simulink model "VRSimulationModel"  (R2020b)
settings: Solver=VariableStepAuto  StartTime=0.0  StopTime=30  RelTol=1e-3
undefined symbols (not defined in the file): cz_length, lane_width
libraries: drivingvehiclecontroller x4, etargetslib x2, rllib x2, dspnetwork x2
settings Model: EnablePacing=on  Creator=ZHANG Meng  LastModifiedBy=ZHANG Meng

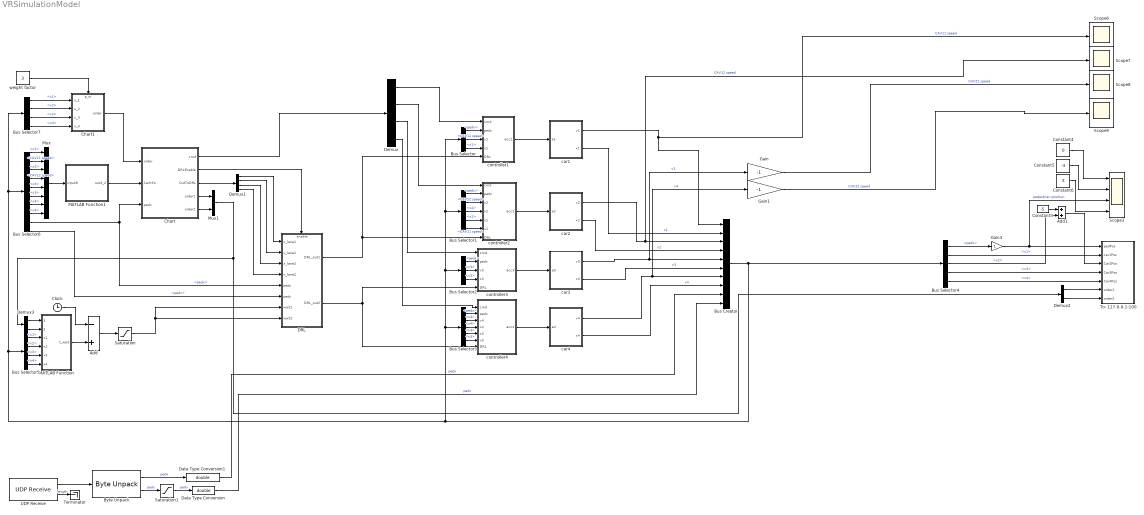
== system VRSimulationModel ==
  Add : Sum  Inputs=-+
  Add1 : Sum
  Bus Creator : BusCreator  Inputs=10
  Bus Selector : BusSelector  OutputSignals=pedx,CAV11 speed,x1
  Bus Selector1 : BusSelector  OutputSignals=pedx,CAV12 speed,x2,x1,CAV11 speed
  Bus Selector2 : BusSelector  OutputSignals=pedx,v3,x3
  Bus Selector3 : BusSelector  OutputSignals=pedx,v4,x4,x3,v3
  Bus Selector4 : BusSelector  OutputSignals=pedx,x1,x2,x3,x4
  Bus Selector5 : BusSelector  OutputSignals=x1,x2,x3,x4
  Bus Selector6 : BusSelector  OutputSignals=x1,CAV11 speed,x2,CAV12 speed,x3,v3,x4,v4,pedx,pedv
  Bus Selector7 : BusSelector  OutputSignals=x1,x2,x3,x4
  Byte Unpack : etargetslib/Byte Unpack  dimensions={1,1}  datatypes={'single','single'}  byteAlign=1
  Chart : Stateflow chart  TreatAsAtomicUnit=on
  Chart1 : Stateflow chart  TreatAsAtomicUnit=on
      settings: PortSchema="{\"entries\":[{\"content\":{\"sides\":[{\"content\":{\"connectorIds\":[\"In1\",\"In2\",\"In3\",\"In4\"]},\"type\":\"ConnectorPlacement.EquallySpacedRectSide\",\"uuid\":\"8a846dc3-1f93-46d5-8c0a-752417c681d9\"},{\"content\":{\"connectorIds\":[\"Out1\"],\"side\":\"RIGHT\"},\"type\":\"ConnectorPlacement.EquallySpacedRectSide\",\"uuid\":\"76ec7057-478a-4564-adde-c35c4c2d4bf9\"},{\"content\":{\"connectorIds\":[\"In5\"],\"side\":\"TOP\"},\"type\":\"ConnectorPlacement.EquallySpacedRectSide\",\"uuid\":\"bd3b034c-69d7-410c-9bea-d641b8557378\"}]},\"type\":\"ConnectorPlacement.EquallySpacedConnector\",\"uuid\":\"e6d2d864-1dd5-4aa2-85d9-3c27811e9247\"}],\"packageUris\":[\"http://schema.mathworks.com/mf0/Connector/R2020b\"],\"version\":\"1.0\"}"
  Clock : Clock
  Constant3 : Constant  Value=-5
  Constant4 : Constant  Value=0
  Constant5 : Constant  Value=-3
  Constant6 : Constant  Value=3
  DRL : Subsystem  TreatAsAtomicUnit=on
  Data Type Conversion : DataTypeConversion  OutDataTypeStr=double
  Data Type Conversion1 : DataTypeConversion  OutDataTypeStr=double
  Demux : Demux
  Demux1 : Demux
  Demux2 : Demux  Outputs=2
  Demux3 : Demux  Outputs=2
  Gain : Gain  Gain=-1
  Gain1 : Gain  Gain=-1
  Gain3 : Gain
  MATLAB Function : MATLAB Function  TreatAsAtomicUnit=on
  MATLAB Function1 : MATLAB Function  TreatAsAtomicUnit=on
  Mux : Mux  Inputs=8
  Mux1 : Mux  Inputs=2
  Saturation : Saturate  UpperLimit=20  LowerLimit=0
  Saturation1 : Saturate  UpperLimit=2  LowerLimit=0
  Scope3 : Scope  NumInputPorts=4
  Scope{6..9} (4 alike) : Scope
  Terminator : Terminator
  To: 127.0.0.1:100 : Subsystem
  UDP Receive : dspnetwork/UDP Receive  localURL='0.0.0.0'  localPort=200  remoteURL='127.0.0.1'  remotePort=-1  recvBufferSize=100  dims=8  signalDatatype=uint8  isComplex=off  isVarSize=off  showBlockingTime=off  blockingTime=0  sampletime=0.1  blockPlatform=[]
  car1 : Subsystem
  car2 : Subsystem
  car3 : Subsystem
  car4 : Subsystem
  controller1 : Subsystem
  controller2 : Subsystem
  controller3 : Subsystem
  controller4 : Subsystem
  weight factor : Constant  Value=3
  wires:
  controller4/1(acc4) -> car4/1(a4)
  controller2/1(acc2) -> car2/1(a2)
  controller3/1(acc3) -> car3/1(a3)
  car1/1(v1) -> Scope6/1, Bus Creator/1  "CAV11 speed"
  car1/2(x1) -> Bus Creator/2  "x1"
  car2/1(v2) -> Scope7/1, Bus Creator/3  "CAV12 speed"
  car2/2(x2) -> Bus Creator/4  "x2"
  car3/1(v3) -> Gain/1, Bus Creator/5  "v3"
  car3/2(x3) -> Bus Creator/6  "x3"
  car4/1(v4) -> Gain1/1, Bus Creator/7  "v4"
  car4/2(x4) -> Bus Creator/8  "x4"
  Bus Creator/1 -> Bus Selector4/1, Bus Selector1/1, Bus Selector/1, Bus Selector2/1, Bus Selector3/1, Bus Selector7/1, Bus Selector6/1, Bus Selector5/1
  Bus Selector/2 -> controller1/3(v1)  "<CAV11 speed>"
  Bus Selector/1 -> controller1/2(pedx)  "<pedx>"
  Bus Selector/3 -> controller1/4(x1)  "<x1>"
  Bus Selector1/5 -> controller2/6(v1)  "<CAV11 speed>"
  Bus Selector1/4 -> controller2/5(x1)  "<x1>"
  Bus Selector1/3 -> controller2/4(x2)  "<x2>"
  Bus Selector1/2 -> controller2/3(v2)  "<CAV12 speed>"
  Bus Selector1/1 -> controller2/2(pedx)  "<pedx>"
  Bus Selector2/1 -> controller3/2(pedx)  "<pedx>"
  Bus Selector2/2 -> controller3/3(v3)  "<v3>"
  Bus Selector2/3 -> controller3/4(x3)  "<x3>"
  Bus Selector3/1 -> controller4/2(pedx)  "<pedx>"
  Bus Selector3/2 -> controller4/3(v4)  "<v4>"
  Bus Selector3/3 -> controller4/4(x4)  "<x4>"
  Bus Selector3/4 -> controller4/5(x3)  "<x3>"
  Bus Selector3/5 -> controller4/6(v3)  "<v3>"
  Demux/4 -> controller4/1(cmd)
  Gain/1 -> Scope8/1  "CAV21 speed"
  Demux/2 -> controller2/1(cmd)
  Gain1/1 -> Scope9/1  "CAV22 speed"
  Demux/3 -> controller3/1(cmd)
  Demux/1 -> controller1/1(cmd)
  Chart/1(cmd) -> Demux/1
  Bus Selector6/8 -> Mux/8  "<v4>"
  Bus Selector6/7 -> Mux/7  "<x4>"
  Bus Selector6/5 -> Mux/5  "<x3>"
  Bus Selector6/6 -> Mux/6  "<v3>"
  Bus Selector6/4 -> Mux/4  "<CAV12 speed>"
  Bus Selector6/3 -> Mux/3  "<x2>"
  Bus Selector6/2 -> Mux/2  "<CAV11 speed>"
  Bus Selector6/1 -> Mux/1  "<x1>"
  Mux/1 -> MATLAB Function1/1(input8)
  MATLAB Function1/1(out4_2) -> Chart/2(CarInfo)
  Bus Selector6/9 -> DRL/5(pedx), Chart/3(pedx)  "<pedx>"
  Chart/3(OutToDRL) -> Demux1/1
  Chart/2(DRLEnable) -> DRL/Enable
  Demux1/1 -> DRL/1(x_lane1)
  Demux1/2 -> DRL/2(v_lane1)
  Demux1/3 -> DRL/3(x_lane2)
  Demux1/4 -> DRL/4(v_lane2)
  Bus Selector6/10 -> DRL/6(pedv)  "<pedv>"
  Bus Selector7/1 -> Chart1/1(x_1)  "<x1>"
  Bus Selector7/2 -> Chart1/2(x_2)  "<x2>"
  Bus Selector7/3 -> Chart1/3(x_3)  "<x3>"
  Bus Selector7/4 -> Chart1/4(x_4)  "<x4>"
  Chart1/1(order) -> Chart/1(order)
  weight factor/1 -> Chart1/5(p_w)
  controller1/1(acc1) -> car1/1(a1)
  DRL/1(DRL_out1) -> controller2/7(DRL), controller1/5(DRL)
  DRL/2(DRL_out2) -> controller4/7(DRL), controller3/5(DRL)
  Saturation/1 -> DRL/7(wait1), DRL/8(wait2)
  Add/1 -> Saturation/1
  MATLAB Function/1(t_wait) -> Add/2
  Clock/1 -> Add/1
  Gain3/1 -> Scope3/3, To: 127.0.0.1:100/1(pedPos)  "pedestrian position"
  Bus Selector4/1 -> Gain3/1  "<pedx>"
  Bus Selector4/5 -> To: 127.0.0.1:100/5(Car4Pos)  "<x4>"
  Constant4/1 -> Scope3/1
  Constant5/1 -> Scope3/2
  Constant6/1 -> Scope3/4
  Chart/4(order1) -> Mux1/1
  Chart/5(order2) -> Mux1/2
  Demux2/1 -> To: 127.0.0.1:100/6(order1)
  Demux2/2 -> To: 127.0.0.1:100/7(order2)
  Mux1/1 -> Demux3/1, Demux2/1
  UDP Receive/1 -> Byte Unpack/1
  Saturation1/1 -> Data Type Conversion/1  "pedv"
  Data Type Conversion1/1 -> Bus Creator/9  "pedx"
  Data Type Conversion/1 -> Bus Creator/10  "pedv"
  Bus Selector5/1 -> MATLAB Function/3(x1)  "<x1>"
  Bus Selector5/2 -> MATLAB Function/4(x2)  "<x2>"
  Bus Selector5/3 -> MATLAB Function/5(x3)  "<x3>"
  Bus Selector5/4 -> MATLAB Function/6(x4)  "<x4>"
  Demux3/1 -> MATLAB Function/1(order1)
  Demux3/2 -> MATLAB Function/2(order2)
  Constant3/1 -> Add1/1
  Bus Selector4/2 -> To: 127.0.0.1:100/2(car1Pos)  "<x1>"
  Bus Selector4/4 -> To: 127.0.0.1:100/4(Car3Pos)  "<x3>"
  Bus Selector4/3 -> Add1/2  "<x2>"
  Add1/1 -> To: 127.0.0.1:100/3(Car2Pos)
  UDP Receive/2 -> Terminator/1  "length"
  Byte Unpack/1 -> Data Type Conversion1/1  "pedx"
  Byte Unpack/2 -> Saturation1/1  "pedv"

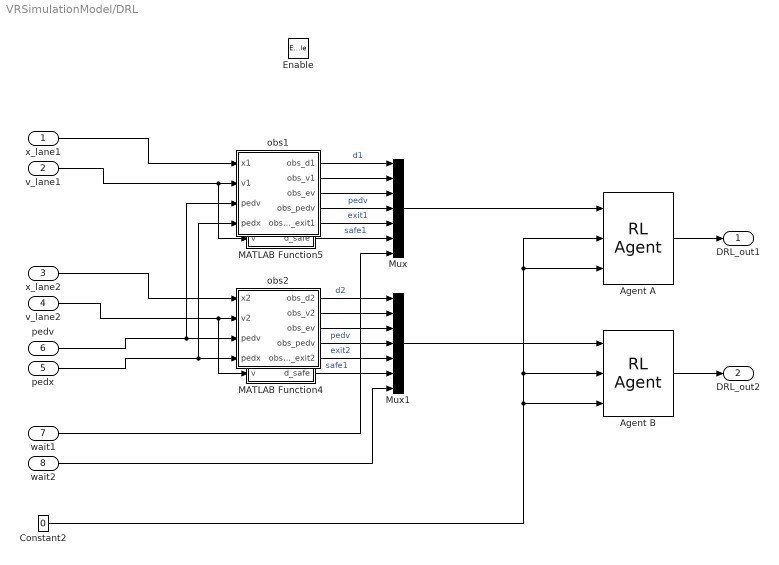
== system VRSimulationModel/DRL ==
  x_lane1 : Inport
  v_lane1 : Inport  Port=2
  x_lane2 : Inport  Port=3
  v_lane2 : Inport  Port=4
  pedx : Inport  Port=5
  pedv : Inport  Port=6
  wait1 : Inport  Port=7
  wait2 : Inport  Port=8
  Enable : EnablePort
  Agent A : rllib/RL Agent  Agent=agentA  ProvideReward=on  ProvideIsDone=on  ProvideCumRwd=off  TreatAsDirectFeedthrough=on  CollectLoggedSignals=on  CollectModelStates=on
  Agent B : rllib/RL Agent  Agent=agentB  ProvideReward=on  ProvideIsDone=on  ProvideCumRwd=off  TreatAsDirectFeedthrough=on  CollectLoggedSignals=on  CollectModelStates=on
  Constant2 : Constant  Value=0
  MATLAB Function4 : MATLAB Function  TreatAsAtomicUnit=on
  MATLAB Function5 : MATLAB Function  TreatAsAtomicUnit=on
  Mux : Mux  Inputs=7
  Mux1 : Mux  Inputs=7
  obs1 : Subsystem
  obs2 : Subsystem
  DRL_out1 : Outport
  DRL_out2 : Outport  Port=2
  wires:
  Constant2/1 -> Agent A/2, Agent A/3, Agent B/2, Agent B/3
  x_lane1/1 -> obs1/1(x1)
  x_lane2/1 -> obs2/1(x2)
  v_lane1/1 -> MATLAB Function5/1(v), obs1/2(v1)
  pedx/1 -> obs1/4(pedx), obs2/4(pedx)
  pedv/1 -> obs1/3(pedv), obs2/3(pedv)
  Agent B/1 -> DRL_out2/1
  Agent A/1 -> DRL_out1/1
  v_lane2/1 -> MATLAB Function4/1(v), obs2/2(v2)
  obs1/1(obs_d1) -> Mux/1  "d1"
  obs1/2(obs_v1) -> Mux/2
  obs1/3(obs_ev) -> Mux/3
  obs1/4(obs_pedv) -> Mux/4  "pedv"
  obs1/5(obs_d_exit1) -> Mux/5  "exit1"
  MATLAB Function5/1(d_safe) -> Mux/6  "safe1"
  obs2/2(obs_v2) -> Mux1/2
  obs2/4(obs_pedv) -> Mux1/4  "pedv"
  obs2/3(obs_ev) -> Mux1/3
  obs2/1(obs_d2) -> Mux1/1  "d2"
  obs2/5(obs_d_exit2) -> Mux1/5  "exit2"
  MATLAB Function4/1(d_safe) -> Mux1/6  "safe1"
  Mux/1 -> Agent A/1
  Mux1/1 -> Agent B/1
  wait1/1 -> Mux/7
  wait2/1 -> Mux1/7

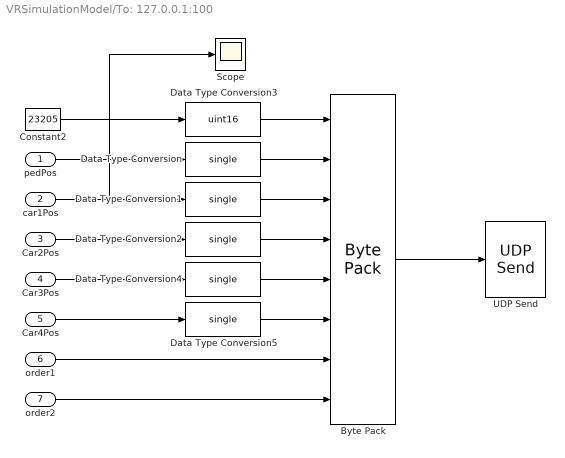
== system VRSimulationModel/To: 127.0.0.1:100 ==
  pedPos : Inport
  car1Pos : Inport  Port=2
  Car2Pos : Inport  Port=3
  Car3Pos : Inport  Port=4
  Car4Pos : Inport  Port=5
  order1 : Inport  Port=6
  order2 : Inport  Port=7
  Byte Pack : etargetslib/Byte Pack  datatypes={'uint16','single','single','single','single','single','uint8','uint8'}  byteAlign=1
  Constant2 : Constant  Value=23205  SampleTime=0.02
  Data Type Conversion{,1..2,4..5} (5 alike) : DataTypeConversion  OutDataTypeStr=single
  Data Type Conversion3 : DataTypeConversion  OutDataTypeStr=uint16
  Scope : Scope
  UDP Send : dspnetwork/UDP Send  remoteURL='127.0.0.1'  remotePort=100  localURL='0.0.0.0'  localPortSource=Specify via dialog  localPort=300  sendBufferSize=200  sampletime=-1  blockPlatform=[]  separateLengthPort=0
  wires:
  Data Type Conversion3/1 -> Byte Pack/1
  Byte Pack/1 -> UDP Send/1
  Constant2/1 -> Data Type Conversion3/1
  car1Pos/1 -> Scope/1, Data Type Conversion1/1
  Data Type Conversion1/1 -> Byte Pack/3
  Data Type Conversion/1 -> Byte Pack/2
  Data Type Conversion2/1 -> Byte Pack/4
  pedPos/1 -> Data Type Conversion/1
  Car2Pos/1 -> Data Type Conversion2/1
  Car4Pos/1 -> Data Type Conversion5/1
  Car3Pos/1 -> Data Type Conversion4/1
  Data Type Conversion4/1 -> Byte Pack/5
  Data Type Conversion5/1 -> Byte Pack/6
  order1/1 -> Byte Pack/7
  order2/1 -> Byte Pack/8

== system VRSimulationModel/car1 ==
  a1 : Inport
  Integrator : Integrator  InitialCondition=10  LimitOutput=on  LowerSaturationLimit=0
  Integrator1 : Integrator  InitialCondition=-30
  Transfer Fcn : TransferFcn  Denominator=[0.2 1]
  v1 : Outport
  x1 : Outport  Port=2
  wires:
  a1/1 -> Transfer Fcn/1
  Integrator/1 -> v1/1, Integrator1/1
  Transfer Fcn/1 -> Integrator/1
  Integrator1/1 -> x1/1

== system VRSimulationModel/car2 ==
  a2 : Inport
  Integrator : Integrator  InitialCondition=10  LimitOutput=on  LowerSaturationLimit=0
  Integrator1 : Integrator  InitialCondition=-75
  Transfer Fcn : TransferFcn  Denominator=[0.2 1]
  v2 : Outport
  x2 : Outport  Port=2
  wires:
  a2/1 -> Transfer Fcn/1
  Integrator/1 -> v2/1, Integrator1/1
  Transfer Fcn/1 -> Integrator/1
  Integrator1/1 -> x2/1

== system VRSimulationModel/car3 ==
  a3 : Inport
  Integrator : Integrator  InitialCondition=-10  LimitOutput=on  UpperSaturationLimit=0
  Integrator1 : Integrator  InitialCondition=35
  Transfer Fcn : TransferFcn  Denominator=[0.2 1]
  v3 : Outport
  x3 : Outport  Port=2
  wires:
  Transfer Fcn/1 -> Integrator/1
  Integrator1/1 -> x3/1
  a3/1 -> Transfer Fcn/1
  Integrator/1 -> v3/1, Integrator1/1

== system VRSimulationModel/car4 ==
  a4 : Inport
  Integrator : Integrator  InitialCondition=-10  LimitOutput=on  UpperSaturationLimit=0
  Integrator1 : Integrator  InitialCondition=70
  Transfer Fcn : TransferFcn  Denominator=[0.2 1]
  v4 : Outport
  x4 : Outport  Port=2
  wires:
  Transfer Fcn/1 -> Integrator/1
  Integrator1/1 -> x4/1
  a4/1 -> Transfer Fcn/1
  Integrator/1 -> v4/1, Integrator1/1

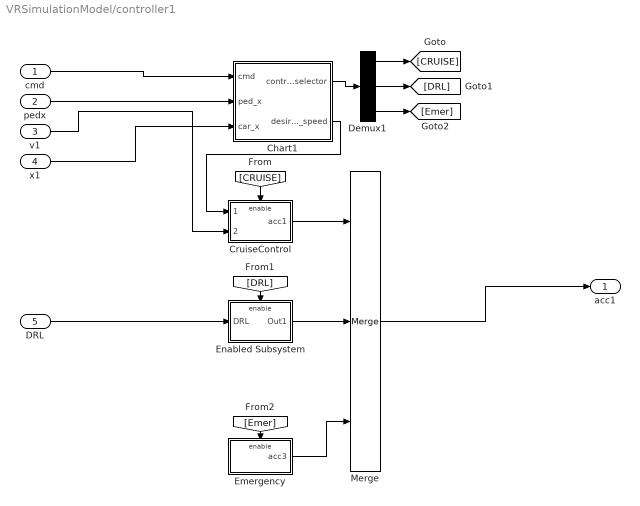
== system VRSimulationModel/controller1 ==
  cmd : Inport
  pedx : Inport  Port=2
  v1 : Inport  Port=3
  x1 : Inport  Port=4
  DRL : Inport  Port=5
  Chart1 : Stateflow chart  TreatAsAtomicUnit=on
  CruiseControl : Subsystem  TreatAsAtomicUnit=on
  Demux1 : Demux  Outputs=3
  Emergency : Subsystem  TreatAsAtomicUnit=on
  Enabled Subsystem : Subsystem  TreatAsAtomicUnit=on
  Merge : Merge  Inputs=3
  acc1 : Outport
  wires:
  [DRL] -> Enabled Subsystem/Enable
  [Emer] -> Emergency/Enable
  Demux1/2 -> [DRL]
  CruiseControl/1(acc1) -> Merge/1
  Demux1/1 -> [CRUISE]
  Demux1/3 -> [Emer]
  [CRUISE] -> CruiseControl/Enable
  Chart1/2(desired_speed) -> CruiseControl/1(RefVelocity)
  Chart1/1(controller_selector) -> Demux1/1
  Merge/1 -> acc1/1
  Emergency/1(acc3) -> Merge/3
  cmd/1 -> Chart1/1(cmd)
  x1/1 -> Chart1/3(car_x)
  Enabled Subsystem/1(Out1) -> Merge/2
  pedx/1 -> Chart1/2(ped_x)
  v1/1 -> CruiseControl/2(CurrVelocity)
  DRL/1 -> Enabled Subsystem/1(DRL)

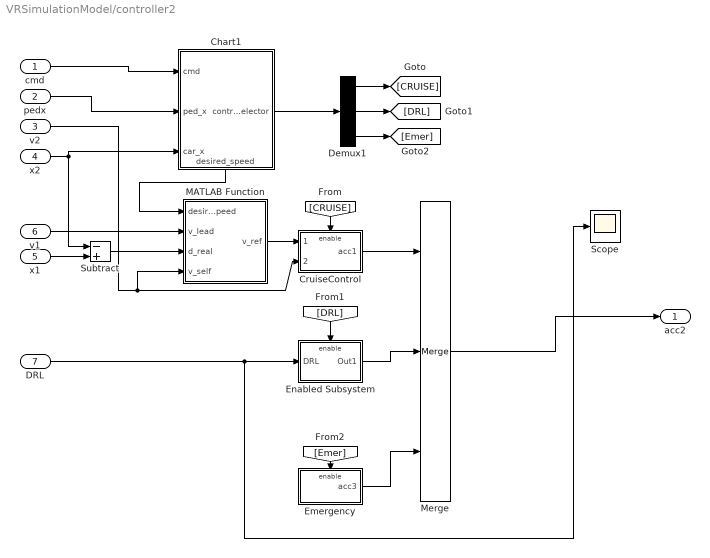
== system VRSimulationModel/controller2 ==
  cmd : Inport
  pedx : Inport  Port=2
  v2 : Inport  Port=3
  x2 : Inport  Port=4
  x1 : Inport  Port=5
  v1 : Inport  Port=6
  DRL : Inport  Port=7
  Chart1 : Stateflow chart  TreatAsAtomicUnit=on
      settings: PortSchema="{\"entries\":[{\"content\":{\"sides\":[{\"content\":{\"connectorIds\":[\"In1\",\"In2\",\"In3\"]},\"type\":\"ConnectorPlacement.EquallySpacedRectSide\",\"uuid\":\"455bd830-a1ef-4c86-a39e-ffcd744a214a\"},{\"content\":{\"connectorIds\":[\"Out1\"],\"side\":\"RIGHT\"},\"type\":\"ConnectorPlacement.EquallySpacedRectSide\",\"uuid\":\"1375661e-f65f-4def-9293-a9836a9e5dc7\"},{\"content\":{\"connectorIds\":[],\"side\":\"TOP\"},\"type\":\"ConnectorPlacement.EquallySpacedRectSide\",\"uuid\":\"6caa9e04-875c-47a2-af51-ebfa3d8838d1\"},{\"content\":{\"connectorIds\":[\"Out2\"],\"side\":\"BOTTOM\"},\"type\":\"ConnectorPlacement.EquallySpacedRectSide\",\"uuid\":\"24a8f513-1368-4415-907e-d61f2bf54b02\"}]},\"type\":\"ConnectorPlacement.EquallySpacedConnector\",\"uuid\":\"c470475d-ef3e-4595-bf6c-24263aaaa3c0\"}],\"packageUris\":[\"http://schema.mathworks.com/mf0/Connector/19700101\"],\"version\":\"1.0\"}"
  CruiseControl : Subsystem  TreatAsAtomicUnit=on
  Demux1 : Demux  Outputs=3
  Emergency : Subsystem  TreatAsAtomicUnit=on
  Enabled Subsystem : Subsystem  TreatAsAtomicUnit=on
  MATLAB Function : MATLAB Function  TreatAsAtomicUnit=on
  Merge : Merge  Inputs=3
  Scope : Scope
  Subtract : Sum  Inputs=-+
  acc2 : Outport
  wires:
  Enabled Subsystem/1(Out1) -> Merge/2
  [DRL] -> Enabled Subsystem/Enable
  [Emer] -> Emergency/Enable
  Demux1/2 -> [DRL]
  CruiseControl/1(acc1) -> Merge/1
  Demux1/1 -> [CRUISE]
  Demux1/3 -> [Emer]
  [CRUISE] -> CruiseControl/Enable
  Chart1/1(controller_selector) -> Demux1/1
  Merge/1 -> acc2/1
  Emergency/1(acc3) -> Merge/3
  v2/1 -> MATLAB Function/4(v_self), CruiseControl/2(CurrVelocity)
  cmd/1 -> Chart1/1(cmd)
  pedx/1 -> Chart1/2(ped_x)
  x2/1 -> Chart1/3(car_x), Subtract/1
  MATLAB Function/1(v_ref) -> CruiseControl/1(RefVelocity)
  Subtract/1 -> MATLAB Function/3(d_real)
  x1/1 -> Subtract/2
  v1/1 -> MATLAB Function/2(v_lead)
  Chart1/2(desired_speed) -> MATLAB Function/1(desired_speed)
  DRL/1 -> Scope/1, Enabled Subsystem/1(DRL)

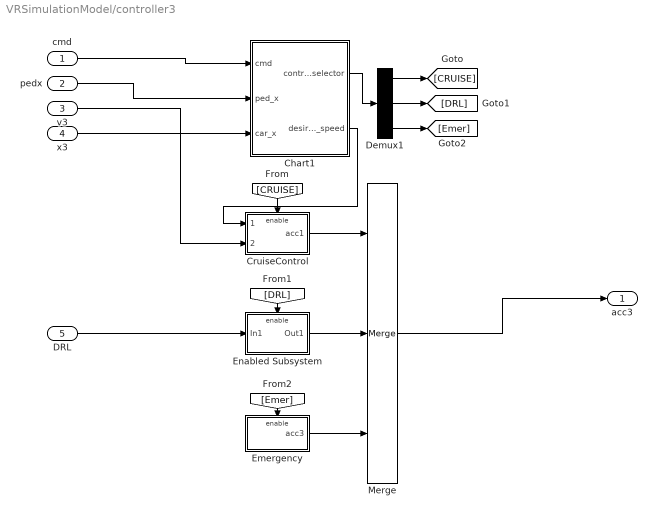
== system VRSimulationModel/controller3 ==
  cmd : Inport
  pedx : Inport  Port=2
  v3 : Inport  Port=3
  x3 : Inport  Port=4
  DRL : Inport  Port=5
  Chart1 : Stateflow chart  TreatAsAtomicUnit=on
  CruiseControl : Subsystem  TreatAsAtomicUnit=on
  Demux1 : Demux  Outputs=3
  Emergency : Subsystem  TreatAsAtomicUnit=on
  Enabled Subsystem : Subsystem  TreatAsAtomicUnit=on
  Merge : Merge  Inputs=3
  acc3 : Outport
  wires:
  [DRL] -> Enabled Subsystem/Enable
  [Emer] -> Emergency/Enable
  Demux1/2 -> [DRL]
  CruiseControl/1(acc1) -> Merge/1
  Demux1/1 -> [CRUISE]
  Demux1/3 -> [Emer]
  [CRUISE] -> CruiseControl/Enable
  Chart1/2(desired_speed) -> CruiseControl/1(RefVelocity)
  Chart1/1(controller_selector) -> Demux1/1
  Merge/1 -> acc3/1
  Emergency/1(acc3) -> Merge/3
  cmd/1 -> Chart1/1(cmd)
  x3/1 -> Chart1/3(car_x)
  Enabled Subsystem/1(Out1) -> Merge/2
  pedx/1 -> Chart1/2(ped_x)
  v3/1 -> CruiseControl/2(CurrVelocity)
  DRL/1 -> Enabled Subsystem/1(In1)

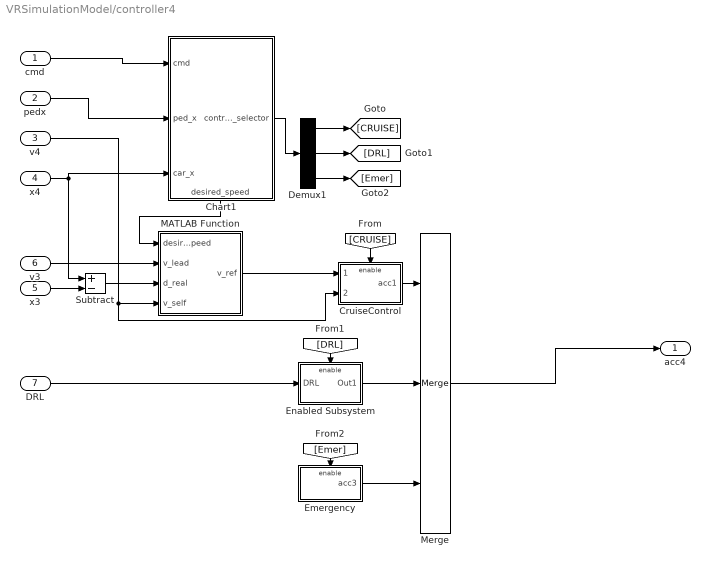
== system VRSimulationModel/controller4 ==
  cmd : Inport
  pedx : Inport  Port=2
  v4 : Inport  Port=3
  x4 : Inport  Port=4
  x3 : Inport  Port=5
  v3 : Inport  Port=6
  DRL : Inport  Port=7
  Chart1 : Stateflow chart  TreatAsAtomicUnit=on
      settings: PortSchema="{\"entries\":[{\"content\":{\"sides\":[{\"content\":{\"connectorIds\":[\"In1\",\"In2\",\"In3\"]},\"type\":\"ConnectorPlacement.EquallySpacedRectSide\",\"uuid\":\"455bd830-a1ef-4c86-a39e-ffcd744a214a\"},{\"content\":{\"connectorIds\":[\"Out1\"],\"side\":\"RIGHT\"},\"type\":\"ConnectorPlacement.EquallySpacedRectSide\",\"uuid\":\"1375661e-f65f-4def-9293-a9836a9e5dc7\"},{\"content\":{\"connectorIds\":[],\"side\":\"TOP\"},\"type\":\"ConnectorPlacement.EquallySpacedRectSide\",\"uuid\":\"6caa9e04-875c-47a2-af51-ebfa3d8838d1\"},{\"content\":{\"connectorIds\":[\"Out2\"],\"side\":\"BOTTOM\"},\"type\":\"ConnectorPlacement.EquallySpacedRectSide\",\"uuid\":\"579f8298-37e8-43e1-bb2a-74855a782830\"}]},\"type\":\"ConnectorPlacement.EquallySpacedConnector\",\"uuid\":\"c470475d-ef3e-4595-bf6c-24263aaaa3c0\"}],\"packageUris\":[\"http://schema.mathworks.com/mf0/Connector/19700101\"],\"version\":\"1.0\"}"
  CruiseControl : Subsystem  TreatAsAtomicUnit=on
  Demux1 : Demux  Outputs=3
  Emergency : Subsystem  TreatAsAtomicUnit=on
  Enabled Subsystem : Subsystem  TreatAsAtomicUnit=on
  MATLAB Function : MATLAB Function  TreatAsAtomicUnit=on
  Merge : Merge  Inputs=3
  Subtract : Sum  Inputs=+-
  acc4 : Outport
  wires:
  Enabled Subsystem/1(Out1) -> Merge/2
  [DRL] -> Enabled Subsystem/Enable
  [Emer] -> Emergency/Enable
  Demux1/2 -> [DRL]
  CruiseControl/1(acc1) -> Merge/1
  Demux1/1 -> [CRUISE]
  Demux1/3 -> [Emer]
  [CRUISE] -> CruiseControl/Enable
  Chart1/1(controller_selector) -> Demux1/1
  Merge/1 -> acc4/1
  Emergency/1(acc3) -> Merge/3
  v4/1 -> MATLAB Function/4(v_self), CruiseControl/2(CurrVelocity)
  cmd/1 -> Chart1/1(cmd)
  pedx/1 -> Chart1/2(ped_x)
  x4/1 -> Chart1/3(car_x), Subtract/1
  MATLAB Function/1(v_ref) -> CruiseControl/1(RefVelocity)
  Subtract/1 -> MATLAB Function/3(d_real)
  x3/1 -> Subtract/2
  v3/1 -> MATLAB Function/2(v_lead)
  Chart1/2(desired_speed) -> MATLAB Function/1(desired_speed)
  DRL/1 -> Enabled Subsystem/1(DRL)

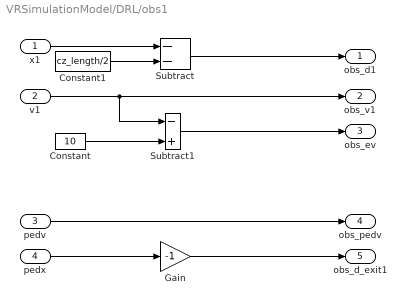
== system VRSimulationModel/DRL/obs1 ==
  x1 : Inport
  v1 : Inport  Port=2
  pedv : Inport  Port=3
  pedx : Inport  Port=4
  Constant : Constant  Value=10
  Constant1 : Constant  Value=cz_length/2
  Gain : Gain  Gain=-1
  Subtract : Sum  Inputs=--
  Subtract1 : Sum  Inputs=-+
  obs_d1 : Outport
  obs_v1 : Outport  Port=2
  obs_ev : Outport  Port=3
  obs_pedv : Outport  Port=4
  obs_d_exit1 : Outport  Port=5
  wires:
  x1/1 -> Subtract/1
  Subtract/1 -> obs_d1/1
  Constant1/1 -> Subtract/2
  v1/1 -> Subtract1/1, obs_v1/1
  pedx/1 -> Gain/1
  pedv/1 -> obs_pedv/1
  Gain/1 -> obs_d_exit1/1
  Constant/1 -> Subtract1/2
  Subtract1/1 -> obs_ev/1

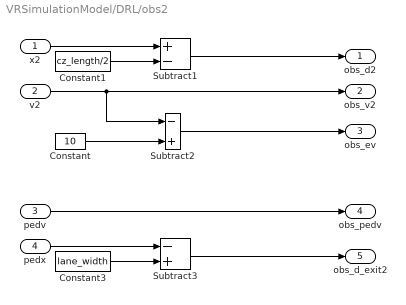
== system VRSimulationModel/DRL/obs2 ==
  x2 : Inport
  v2 : Inport  Port=2
  pedv : Inport  Port=3
  pedx : Inport  Port=4
  Constant : Constant  Value=10
  Constant1 : Constant  Value=cz_length/2
  Constant3 : Constant  Value=lane_width
  Subtract1 : Sum  Inputs=+-
  Subtract2 : Sum  Inputs=-+
  Subtract3 : Sum  Inputs=-+
  obs_d2 : Outport
  obs_v2 : Outport  Port=2
  obs_ev : Outport  Port=3
  obs_pedv : Outport  Port=4
  obs_d_exit2 : Outport  Port=5
  wires:
  Constant1/1 -> Subtract1/2
  x2/1 -> Subtract1/1
  Subtract1/1 -> obs_d2/1
  pedx/1 -> Subtract3/1
  pedv/1 -> obs_pedv/1
  Constant3/1 -> Subtract3/2
  Subtract3/1 -> obs_d_exit2/1
  v2/1 -> Subtract2/1, obs_v2/1
  Subtract2/1 -> obs_ev/1
  Constant/1 -> Subtract2/2

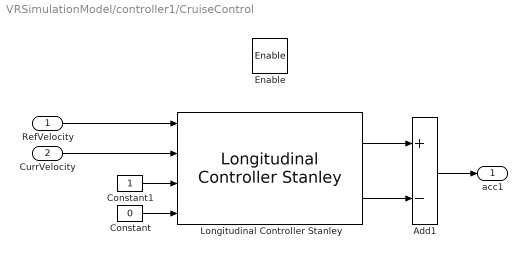
== system VRSimulationModel/controller1/CruiseControl ==
  RefVelocity : Inport
  CurrVelocity : Inport  Port=2
  Enable : EnablePort
  Add1 : Sum  Inputs=+-
  Constant : Constant  Value=0
  Constant1 : Constant
  Longitudinal Controller Stanley : drivingvehiclecontroller/Longitudinal Controller Stanley  Kp=2.5  Ki=1  SampleTime=0.1  MaxAcceleration=2  MaxDeceleration=3
      settings: SourceProductBaseCode=DR
  acc1 : Outport
  wires:
  Longitudinal Controller Stanley/1 -> Add1/1
  Add1/1 -> acc1/1
  Longitudinal Controller Stanley/2 -> Add1/2
  Constant/1 -> Longitudinal Controller Stanley/4
  Constant1/1 -> Longitudinal Controller Stanley/3
  RefVelocity/1 -> Longitudinal Controller Stanley/1
  CurrVelocity/1 -> Longitudinal Controller Stanley/2

== system VRSimulationModel/controller1/Emergency ==
  Enable : EnablePort
  Constant : Constant  Value=-5  SampleTime=0.1
  acc3 : Outport
  wires:
  Constant/1 -> acc3/1

== system VRSimulationModel/controller1/Enabled Subsystem ==
  DRL : Inport
  Enable : EnablePort
  Out1 : Outport  InitialOutput=0  VectorParamsAs1DForOutWhenUnconnected=off
  wires:
  DRL/1 -> Out1/1

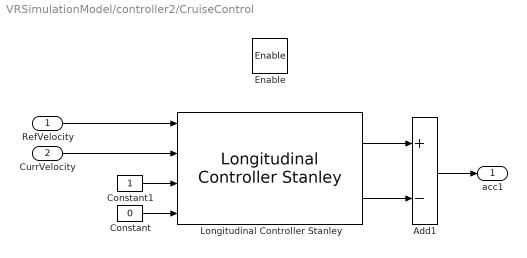
== system VRSimulationModel/controller2/CruiseControl ==
  RefVelocity : Inport
  CurrVelocity : Inport  Port=2
  Enable : EnablePort
  Add1 : Sum  Inputs=+-
  Constant : Constant  Value=0
  Constant1 : Constant
  Longitudinal Controller Stanley : drivingvehiclecontroller/Longitudinal Controller Stanley  Kp=2.5  Ki=1  SampleTime=0.1  MaxAcceleration=2  MaxDeceleration=3
      settings: SourceProductBaseCode=DR
  acc1 : Outport
  wires:
  Longitudinal Controller Stanley/1 -> Add1/1
  Add1/1 -> acc1/1
  Longitudinal Controller Stanley/2 -> Add1/2
  Constant/1 -> Longitudinal Controller Stanley/4
  Constant1/1 -> Longitudinal Controller Stanley/3
  RefVelocity/1 -> Longitudinal Controller Stanley/1
  CurrVelocity/1 -> Longitudinal Controller Stanley/2

== system VRSimulationModel/controller2/Emergency ==
  Enable : EnablePort
  Constant : Constant  Value=-5  SampleTime=0.1
  acc3 : Outport
  wires:
  Constant/1 -> acc3/1

== system VRSimulationModel/controller2/Enabled Subsystem ==
  DRL : Inport
  Enable : EnablePort
  Out1 : Outport  InitialOutput=0  VectorParamsAs1DForOutWhenUnconnected=off
  wires:
  DRL/1 -> Out1/1

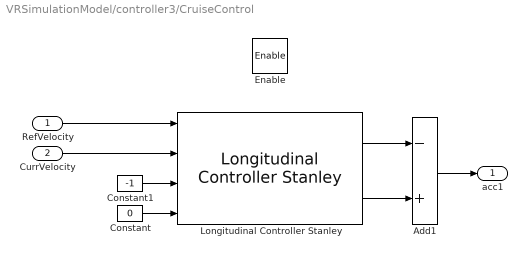
== system VRSimulationModel/controller3/CruiseControl ==
  RefVelocity : Inport
  CurrVelocity : Inport  Port=2
  Enable : EnablePort
  Add1 : Sum  Inputs=-+
  Constant : Constant  Value=0
  Constant1 : Constant  Value=-1
  Longitudinal Controller Stanley : drivingvehiclecontroller/Longitudinal Controller Stanley  Kp=2.5  Ki=1  SampleTime=0.1  MaxAcceleration=2  MaxDeceleration=3
      settings: SourceProductBaseCode=DR
  acc1 : Outport
  wires:
  Longitudinal Controller Stanley/1 -> Add1/1
  Add1/1 -> acc1/1
  Longitudinal Controller Stanley/2 -> Add1/2
  Constant/1 -> Longitudinal Controller Stanley/4
  Constant1/1 -> Longitudinal Controller Stanley/3
  RefVelocity/1 -> Longitudinal Controller Stanley/1
  CurrVelocity/1 -> Longitudinal Controller Stanley/2

== system VRSimulationModel/controller3/Emergency ==
  Enable : EnablePort
  Constant : Constant  Value=5  SampleTime=0.1
  acc3 : Outport
  wires:
  Constant/1 -> acc3/1

== system VRSimulationModel/controller3/Enabled Subsystem ==
  In1 : Inport
  Enable : EnablePort
  Gain : Gain  Gain=-1
  Out1 : Outport  InitialOutput=0  VectorParamsAs1DForOutWhenUnconnected=off
  wires:
  In1/1 -> Gain/1
  Gain/1 -> Out1/1

== system VRSimulationModel/controller4/CruiseControl ==
  RefVelocity : Inport
  CurrVelocity : Inport  Port=2
  Enable : EnablePort
  Add1 : Sum  Inputs=-+
  Constant : Constant  Value=0
  Constant1 : Constant  Value=-1
  Longitudinal Controller Stanley : drivingvehiclecontroller/Longitudinal Controller Stanley  Kp=2.5  Ki=1  SampleTime=0.1  MaxAcceleration=2  MaxDeceleration=3
      settings: SourceProductBaseCode=DR
  acc1 : Outport
  wires:
  Longitudinal Controller Stanley/1 -> Add1/1
  Add1/1 -> acc1/1
  Longitudinal Controller Stanley/2 -> Add1/2
  Constant/1 -> Longitudinal Controller Stanley/4
  Constant1/1 -> Longitudinal Controller Stanley/3
  RefVelocity/1 -> Longitudinal Controller Stanley/1
  CurrVelocity/1 -> Longitudinal Controller Stanley/2

== system VRSimulationModel/controller4/Emergency ==
  Enable : EnablePort
  Constant : Constant  Value=5  SampleTime=0.1
  acc3 : Outport
  wires:
  Constant/1 -> acc3/1

== system VRSimulationModel/controller4/Enabled Subsystem ==
  DRL : Inport
  Enable : EnablePort
  Gain : Gain  Gain=-1
  Out1 : Outport  InitialOutput=0  VectorParamsAs1DForOutWhenUnconnected=off
  wires:
  DRL/1 -> Gain/1
  Gain/1 -> Out1/1

== stateflow chart VRSimulationModel/controller1/Chart1 ==
  state CrossFirst % select cruise
    en: controller_selector = [true;false;false];
    desired_speed = 12; % reference speed
  note: cruise with max speed
  state NormalDriving % select cruise
    en: controller_selector = [true;false;false];
    desired_speed = 10; % reference speed
    du:
  state EmergencyBrake % select emergency brake
    en: controller_selector = [false;false;true];
  note: emergent state
  state WaitPedestrian % select DRL
    en: controller_selector = [false;true;false];
  note: cruise with desired speed
  NormalDriving % select cruise -> CrossFirst % select cruise [order 1] : [cmd == 1 && ped_x < -3 && car_x < 5]
  CrossFirst % select cruise -> NormalDriving % select cruise [order 2] : [car_x > 5]
  CrossFirst % select cruise -> EmergencyBrake % select emergency brake [order 1] : [ped_x > -3 && ped_x < 0]
  (default) -> NormalDriving % select cruise
  EmergencyBrake % select emergency brake -> NormalDriving % select cruise : [ped_x <-3 || ped_x > 0 || car_x>5]
  NormalDriving % select cruise -> WaitPedestrian % select DRL [order 2] : [cmd == 2 && ped_x < 0]
  WaitPedestrian % select DRL -> NormalDriving % select cruise : [ped_x > 0]
  data: controller_selector output boolean size=3; desired_speed output double size=1; cmd input; ped_x input; car_x input

== stateflow chart VRSimulationModel/controller2/Chart1 ==
  state CrossFirst % select cruise
    en: controller_selector = [true;false;false];
    desired_speed = 12;
  state NormalDriving % select cruise
    en: controller_selector = [true;false;false];
    desired_speed = 10;
  note: cruise with max speed
  state EmergencyBrake % select emergency brake
    en: controller_selector = [false;false;true];
  note: emergent state
  state WaitPedestrian % select DRL
    en: controller_selector = [false;true;false];
  note: cruise with desired speed
  state status1 = isNormalDriving(info) [function]
    (default) -> (junction 47) : % normal driving
    (junction 47) -> (junction 48) [order 1] : [info >0 ]
    (junction 47) -> (junction 49) [order 2] : {status1 = false;}
    (junction 48) -> (junction 50) : {status1 = true;}
    (junction 50) -> (junction 49)
    (junction 49) -> (junction 51)
  state status2 = isCrossFirst(info) [function]
    (default) -> (junction 62) : % cross first
    (junction 62) -> (junction 63) [order 1] : [info > 2 && info<4]
    (junction 62) -> (junction 64) [order 2] : {status2 = false;}
    (junction 63) -> (junction 65) : {status2 = true;}
    (junction 65) -> (junction 64)
    (junction 64) -> (junction 66)
  state status3 = isWaiting(info) [function]
    (default) -> (junction 82) : % cross first
    (junction 82) -> (junction 81) [order 1] : [info > 4 && info<6]
    (junction 82) -> (junction 84) [order 2] : {status3 = false;}
    (junction 81) -> (junction 85) : {status3 = true;}
    (junction 85) -> (junction 84)
    (junction 84) -> (junction 80)
  state status4 = isEmergency(info) [function]
    (default) -> (junction 98) : % emergent state
    (junction 98) -> (junction 97) [order 1] : [info > 6 && info<8]
    (junction 98) -> (junction 100) [order 2] : {status4 = false;}
    (junction 97) -> (junction 101) : {status4 = true;}
    (junction 101) -> (junction 100)
    (junction 100) -> (junction 96)
  NormalDriving % select cruise -> CrossFirst % select cruise [order 1] : [cmd == 1 && ped_x < -3 && car_x < 5]
  CrossFirst % select cruise -> NormalDriving % select cruise [order 2] : [car_x > 5]
  CrossFirst % select cruise -> EmergencyBrake % select emergency brake [order 1] : [ped_x > -3 && ped_x < 0]
  (default) -> NormalDriving % select cruise
  EmergencyBrake % select emergency brake -> NormalDriving % select cruise : [ped_x < -3 || ped_x > 0 || car_x>5]
  NormalDriving % select cruise -> WaitPedestrian % select DRL [order 2] : [cmd == 2 && ped_x < 0]
  WaitPedestrian % select DRL -> NormalDriving % select cruise : [ped_x > 0]
  data: info function_input; status1 function_output; info function_input; status2 function_output; info function_input; status3 function_output; info function_input; status4 function_output; controller_selector output boolean size=3; cmd input; ped_x input; car_x input; desired_speed output

== stateflow chart VRSimulationModel/controller3/Chart1 ==
  state CrossFirst % select cruise
    en: controller_selector = [true;false;false];
    desired_speed = -12; % reference speed
  state NormalDriving % select cruise
    en: controller_selector = [true;false;false];
    desired_speed = -10; % reference speed
    du:
  note: cruise with max speed
  state EmergencyBrake % select emergency brake
    en: controller_selector = [false;false;true];
  note: emergent state
  state WaitPedestrian % select DRL
    en: controller_selector = [false;true;false];
  note: cruise with desired speed
  NormalDriving % select cruise -> CrossFirst % select cruise [order 1] : [cmd == 1 && ped_x < 0 && car_x > -5]
  CrossFirst % select cruise -> NormalDriving % select cruise [order 2] : [car_x < -5]
  CrossFirst % select cruise -> EmergencyBrake % select emergency brake [order 1] : [ped_x > 0 && ped_x < 3]
  (default) -> NormalDriving % select cruise
  EmergencyBrake % select emergency brake -> NormalDriving % select cruise : [ped_x < 0 || ped_x > 3 || car_x<-5]
  NormalDriving % select cruise -> WaitPedestrian % select DRL [order 2] : [cmd == 2 && ped_x < 3]
  WaitPedestrian % select DRL -> NormalDriving % select cruise : [ped_x > 3]
  data: controller_selector output boolean size=3; desired_speed output double size=1; cmd input; ped_x input; car_x input

== stateflow chart VRSimulationModel/controller4/Chart1 ==
  state CrossFirst % select cruise
    en: controller_selector = [true;false;false];
    desired_speed = -12;
  state NormalDriving % select cruise
    en: controller_selector = [true;false;false];
    desired_speed = -10;
  note: cruise with max speed
  state EmergencyBrake % select emergency brake
    en: controller_selector = [false;false;true];
  note: emergent state
  state WaitPedestrian % select DRL
    en: controller_selector = [false;true;false];
  note: cruise with desired speed
  NormalDriving % select cruise -> CrossFirst % select cruise [order 1] : [cmd == 1 && ped_x < 0 && car_x > -5]
  CrossFirst % select cruise -> NormalDriving % select cruise [order 2] : [car_x < -5]
  CrossFirst % select cruise -> EmergencyBrake % select emergency brake [order 1] : [ped_x > 0 && ped_x < 3]
  (default) -> NormalDriving % select cruise
  EmergencyBrake % select emergency brake -> NormalDriving % select cruise : [ped_x < 0 || ped_x > 3 || car_x<-5]
  NormalDriving % select cruise -> WaitPedestrian % select DRL [order 2] : [cmd == 2 && ped_x < 3]
  WaitPedestrian % select DRL -> NormalDriving % select cruise : [ped_x > 3]
  data: controller_selector output boolean size=3; cmd input; ped_x input; car_x input; desired_speed output

== matlab function VRSimulationModel/controller2/MATLAB Function ==
  data: desired_speed input; v_lead input; d_real input; v_self input; v_ref output
function v_ref = fcn(desired_speed, v_lead, d_real, v_self)
    d_default = 15;
    t_gap = 1.4;
    v_hat = desired_speed;
    
    d_safe = d_default + t_gap * v_self;
    if d_safe > d_real
        v_ref = min(v_lead, v_hat);
    else
        v_ref = v_hat;
    end
end

== matlab function VRSimulationModel/controller4/MATLAB Function ==
  data: desired_speed input; v_lead input; d_real input; v_self input; v_ref output
function v_ref = fcn(desired_speed, v_lead, d_real, v_self)
    d_default = 15;
    t_gap = 1.4;
    v_hat = desired_speed;
    
    d_safe = d_default + t_gap * (-v_self);
    if d_safe > d_real
        v_ref = max(v_lead, v_hat);
    else
        v_ref = v_hat;
    end
    
end

== matlab function VRSimulationModel/DRL/MATLAB Function4 ==
  data: v input; d_safe output
function d_safe  = SafetyReward(v)
    d_safe = v^2/6 + v;  % needed safe distance for car1
end

== stateflow chart VRSimulationModel/Chart ==
  state State2223
    en:cmd = [2;0;2;0];
    DRLEnable = true;
    du:OutToDRL=[CarInfo(1,1) ...
    CarInfo(1,2) CarInfo(3,1) -CarInfo(3,2)];
  state State2227
    en:cmd = [1;1;1;1]
    DRLEnable = false;
  note: 1
  note: 9
  state State2224
    en:cmd = [1;2;2;0];
    DRLEnable = true;
    du:OutToDRL=[CarInfo(2,1) CarInfo(2,2)...
    CarInfo(3,1) -CarInfo(3,2)];
  state State2226
    en:cmd = [1;2;1;1];
    DRLEnable = true;
    du:OutToDRL=...
    [CarInfo(2,1) CarInfo(2,2) ...
    -CarInfo(2,1) CarInfo(2,2)];
  state InitialState00001
    en: cmd = [0;0;0;0];
    DRLEnable = false;
  note: 2
  note: 8
  state State2225
    en:cmd = [1;1;2;0];
    DRLEnable = true;
    du:OutToDRL = ...
    [-CarInfo(3,1) -CarInfo(3,2) ...
    CarInfo(3,1) -CarInfo(3,2)];
  state State2229
    en:cmd = [1;2;1;2];
    DRLEnable = true;
    du:OutToDRL=[CarInfo(2,1)...
    CarInfo(2,2) CarInfo(4,1)...
    -CarInfo(4,2)];
  state State2230
    en:cmd = [2;0;1;1];
    DRLEnable = true;
    du:OutToDRL=...
    [CarInfo(1,1) CarInfo(1,2)...
    -CarInfo(1,1) CarInfo(1,2)];
  state State2231
    en:cmd = [1;1;1;2];
    DRLEnable = true;
    du:OutToDRL=...
    [-CarInfo(4,1) -CarInfo(4,2) ...
    CarInfo(4,1) -CarInfo(4,2)];
  state State2228
    en:cmd = [2;0;1;2];
    DRLEnable = true;
    du:OutToDRL=[CarInfo(1,1) ...
    CarInfo(1,2) CarInfo(4,1)...
    -CarInfo(4,2)];
  note: 4
  note: 3
  note: 5
  note: 6
  note: 7
  (default) -> InitialState00001
  InitialState00001 -> State2227 [order 1] : [order(1) == 2 && order(2) == 2 && pedx<3]
      | {order1 = 2; order2 = 2}
  InitialState00001 -> State2223 [order 9] : [order(1) == 0 && order(2) == 0&& pedx<3]
      | {order1 = 0; order2 = 0}
  State2223 -> InitialState00001 : [pedx>3]
  State2227 -> InitialState00001 : [pedx>3]
  InitialState00001 -> State2226 [order 3] : [order(1) == 1 && order(2) == 2 && pedx<3]
      | {order1 = 1; order2 = 2}
  InitialState00001 -> State2224 [order 8] : [order(1) == 1 && order(2) == 0 && pedx<3]
      | {order1 = 1; order2 = 0}
  State2224 -> InitialState00001 : [pedx>3]
  State2226 -> InitialState00001 : [pedx>3]
  State2225 -> InitialState00001 : [pedx>3]
  InitialState00001 -> State2230 [order 2] : [order(1) == 0 && order(2) == 2 && pedx<3]
      | {order1 = 0; order2 = 2}
  State2230 -> InitialState00001 : [pedx>3]
  InitialState00001 -> State2225 [order 7] : [order(1) == 2 && order(2) == 0 && pedx<3]
      | {order1 = 2; order2 = 0}
  InitialState00001 -> State2231 [order 4] : [order(1) == 2 && order(2) == 1 && pedx<3]
      | {order1 = 2; order2 = 1}
  State2231 -> InitialState00001 : [pedx>3]
  InitialState00001 -> State2229 [order 5] : [order(1) == 1 && order(2) == 1 && pedx<3]
      | {order1 = 1; order2 = 1}
  State2229 -> InitialState00001 : [pedx>3]
  InitialState00001 -> State2228 [order 6] : [order(1) == 0 && order(2) == 1 && pedx<3]
      | {order1 = 0; order2 = 1}
  State2228 -> InitialState00001 : [pedx>3]
  data: cmd output size=4; order input size=[1 2]; DRLEnable output boolean size=1; CarInfo input size=[4 2]; OutToDRL output size=[1 4]; pedx input; order1 output uint8; order2 output uint8

== matlab function VRSimulationModel/MATLAB Function1 ==
  data: input8 input; out4_2 output
function out4_2 = SignalAssigment(input8)
    out4_2 = [input8(1) input8(2);input8(3) input8(4);input8(5) input8(6);input8(7) input8(8)];
end

== matlab function VRSimulationModel/DRL/MATLAB Function5 ==
  data: v input; d_safe output
function d_safe  = SafetyReward(v)
    d_safe = v^2/6 + v;  % needed safe distance for car1
end

== stateflow chart VRSimulationModel/Chart1 ==
  state orderGenerate
    en: [loss, order] = PassOrderGenerator( [-x_1+5 -x_2+5], [x_3+5 x_4+5], p_w )
  (default) -> orderGenerate
  data: CAVLane1 function_input; CAVLane2 function_input; weightFactorPed function_input; outLoss function_output size=9; outOrder function_output; x_1 input size=1; x_2 input size=1; x_3 input size=1; x_4 input size=1; order output size=[1 2]; p_w input; loss local size=9
  function [outLoss, outOrder]  = PassOrderGenerator(CAVLane1,CAVLane2,weightFactorPed):
    | function [outLoss, outOrder]  = PassOrderGenerator(CAVLane1,CAVLane2,weightFactorPed)
    | %UNTITLED caculate the opimal intersection sequence.
    | %   此处显示详细说明
    | % d_vi_exit = [30 55 100];
    | % d_vj_exit = [30 80 124];
    | 
    | d_vi_exit = CAVLane1;
    | d_vj_exit = CAVLane2;
    | 
    | d_base = 24;
    | %w_p = 5;
    | w_p = weightFactorPed;
    | w_v = 1;
    | 
    | LOSS_rec = 10000;
    | i_rec = 0;
    | j_rec = 0;
    | % pedestrian cross before car_i, car_j
    | m = length(d_vi_exit);
    | n = length(d_vj_exit);
    | result = zeros([(m+1) (n+1)]);
    | for i = 0 : m
    |     for j = 0 : n
    |         if i == 0
    |             t_vi_exit = 0;
    |         else
    |             t_vi_exit = d_vi_exit(i)/10; 
    |         end
    |         if j == 0
    |             t_vj_exit = 0;
    |         else
    |             t_vj_exit = d_vj_exit(j)/10;
    |         end
    |         
    |         t_v_exit = max(t_vi_exit , t_vj_exit);
    |         t_p_wait = t_v_exit +1.2;                 % pedestrian waiting time
    |         p_loss = t_p_wait;
    |         
    |         if i==m
    |             d_loss_a = 0;
    |         else
    |             d_loss_a = (m-i)*( -(d_vi_exit(i+1)-10) + 10*(t_p_wait+(4/1)+4.7/2)-(-10+18));% cause problem.
    |             d_k_sum = 0;
    |             if m-i-1 == 0
    |                 d_k_sum = 0;
    |             else
    |                 for k = 1:m-i-1       % m-i-1>0
    |                     d_k = d_vi_exit(i+1+k) - d_vi_exit(i+k);
    |                     d_k_sum = d_k_sum + d_k;   %跟随避让行人的CAV增加的距离
    |                 end
    |             end
    |             d_loss_a = d_loss_a + (m-i-1)*d_base - d_k_sum;
    |         end
    |         if j==n
    |             d_loss_b = 0;
    |         else
    |             d_loss_b = (n-j)*( -(d_vj_exit(j+1)-10) + 10*(t_p_wait+(8/1)+4.7/2) + (-8));
    |             d_k_sum = 0;   %计算跟随避让行人的CAV增加的距离
    |             if n-j-1 == 0
    |                 d_k_sum = 0;
    |             else
    |                 for k = 1:n-j-1       % m-i-1>0
    |                     d_k = d_vj_exit(j+1+k) - d_vj_exit(j+k);
    |                     d_k_sum = d_k_sum + d_k;   %跟随避让行人的CAV增加的距离
    |                 end
    |             end
    |             d_loss_b = d_loss_b + (n-j-1)*d_base - d_k_sum;    %最终的d_loss_a计入CAV增加的跟随距离
    |         end
    |         
    |         %LOSS = w_p*p_loss + w_v*d_loss_a + w_v*d_loss_b;  % sum of loss;
    |         LOSS = w_p * power(p_loss,2) + w_v*d_loss_a + w_v*d_loss_b;  % sum of loss;
    |         
    |         result(i+1, j+1) = LOSS;
    |         if LOSS < LOSS_rec            
    |             LOSS_rec = LOSS;            
    |             i_rec = i;    
    |             j_rec = j;            
    |         end
    |     end
    | end
    | 
    | %x = 1:(m+1)*(n+1);.
    | y = result(:);
    | % plot(x,y,'--gs',...
    | %     'LineWidth',2,...
    | %     'MarkerSize',10,...
    | %     'MarkerEdgeColor','b',...
    | %     'MarkerFaceColor',[0.5,0.5,0.5]);
    | 
    | outLoss = y;
    | outOrder = [i_rec j_rec];
    | end

== matlab function VRSimulationModel/MATLAB Function ==
  data: order1 input; t_wait output; order2 input; x1 input; x2 input; x3 input; x4 input
function t_wait = fcn(order1,order2,x1,x2,x3,x4)
t_wait=0;
tr=1.5;
x1 = 5-x1;
x2 = 5-x2;
x3 = x3+5;
x4 = x4+5;
if order1 == 0
    if order2 == 0 
        t_wait = 0; 
    end
    if order2 == 1 
        t_wait = x3/11; 
    end
    if order2 == 2 
        t_wait = x4/11; 
    end
end

if order1 == 1
    if order2 == 0 
        t_wait = x1/10; 
    end
    if order2 == 1 
        t_wait = max(x1/10,x3/10); 
    end
    if order2 == 2 
        t_wait = max(x1/10,x4/10); 
    end
end

if order1 == 2
    if order2 == 0 
        t_wait = x2/10; 
    end
    if order2 == 1 
        t_wait = max(x2/10,x3/10); 
    end
    if order2 == 2 
        t_wait = max(x2/10,x4/10); 
    end
end


t_wait = t_wait +tr;
